simulink model "sistemaTruxalCon"  (R2024b)
settings: Solver=VariableStepAuto  StartTime=0.0  StopTime=10.0  RelTol=1e-3
undefined symbols (not defined in the file): step_value, Ts
settings Model: Creator=estel  LastModifiedBy=estel

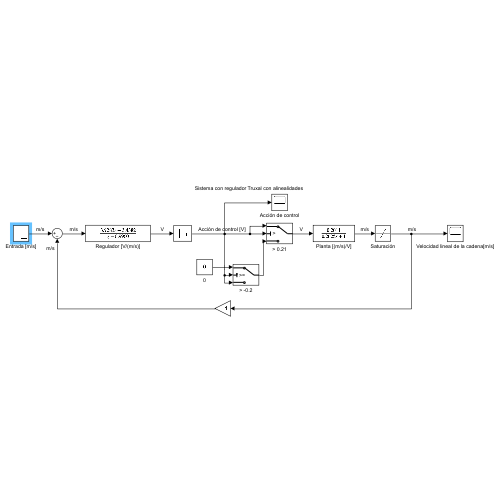
[thumbnail: Simulink's stored preview of the top-level diagram]
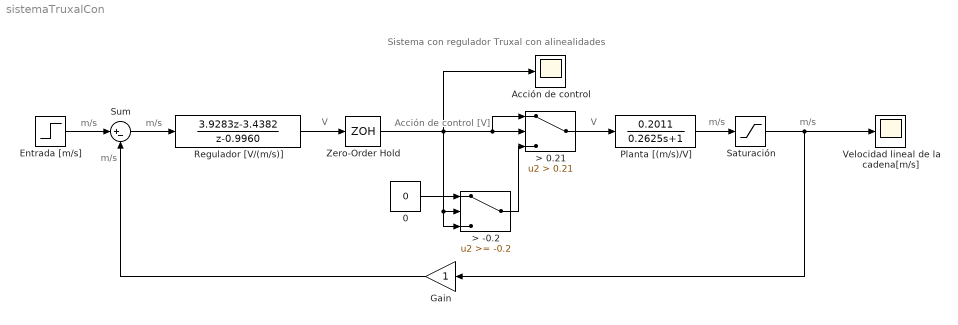
== system sistemaTruxalCon ==
  note: Sistema con regulador Truxal con alinealidades
  note: m/s
  note: m/s
  note: m/s
  note: m/s
  note: V
  note: Acción de control [V]
  note: m/s
  note: V
  0 : Constant  Value=0
  > -0.2 : Switch  Threshold=-0.2  SaturateOnIntegerOverflow=off  InputSameDT=off
  > 0.21 : Switch  Criteria=u2 > Threshold  Threshold=0.21  SaturateOnIntegerOverflow=off  InputSameDT=off
  Acción de control : Scope
  Entrada [m/s] : Step  Time=0  After=step_value  SampleTime=Ts
  Gain : Gain
  Planta [(m/s)/V] : TransferFcn  Numerator=[0.2011]  Denominator=[0.2625 1]
  Regulador [V/(m/s)] : DiscreteTransferFcn  Numerator=[3.9283 -3.4382]  Denominator=[1 -0.9960]
  Saturación : Saturate  UpperLimit=2.1098  LowerLimit=-2.1123
  Sum : Sum  Inputs=|+-
  Velocidad lineal de la cadena[m/s] : Scope
  Zero-Order Hold : ZeroOrderHold  SampleTime=-1
  wires:
  Entrada [m/s]/1 -> Sum/1
  Sum/1 -> Regulador [V/(m/s)]/1
  Gain/1 -> Sum/2
  Regulador [V/(m/s)]/1 -> Zero-Order Hold/1
  0/1 -> > -0.2/1
  > -0.2/1 -> > 0.21/3
  Planta [(m/s)/V]/1 -> Saturación/1
  Saturación/1 -> Gain/1, Velocidad lineal de la cadena[m/s]/1
  > 0.21/1 -> Planta [(m/s)/V]/1
  Zero-Order Hold/1 -> > -0.2/2, > -0.2/3, Acción de control/1, > 0.21/1, > 0.21/2
